simulink model "QuarterCarEKF"  (Simulink 7.5)
settings: Solver=ode45  StartTime=0.0  StopTime=5  FixedStep=0.001  MaxStep=Ts  RelTol=1e-3
PreLoadFcn:
  | QuarterCarParams
values from neighbouring files (symbols this model uses):
  actuatorDelay = 0.005    [QuarterCarParams.m]
  actuatorPole = 70    [QuarterCarParams.m]
  actuatorSat = 4000    [QuarterCarParams.m]
  g = 9.81    [QuarterCarParams.m]
  J = 1    [QuarterCarParams.m]
  Ki = 100000    [QuarterCarParams.m]
  Kp = 1200    [QuarterCarParams.m]
  lambda_ref = 0.1    [QuarterCarParams.m]
  m = 450    [QuarterCarParams.m]
  m0 = m    (= 450)    [QuarterCarParams.m]
  roadCoeffs = [1.28 23.99 0.52]    [QuarterCarParams.m]
  Ts = 0.005    [QuarterCarParams.m]
  v0 = 30    [QuarterCarParams.m]
  Wr = 0.32    [QuarterCarParams.m]
undefined symbols (not defined in the file or in its folder): DiscIntNeverNeededParam
libraries: simulink x3
settings Model: Creator=SIMONE  LastModifiedBy=Phil Goddard
settings DataIOCC: LimitDataPoints=off  SaveOutput=off  SignalLogging=off  DSMLogging=off  SaveTime=off  TimeSaveName=t_out
settings OptimizationCC: InitFltsAndDblsToZero=on
settings DebuggingCC: StrictBusMsg=Warning

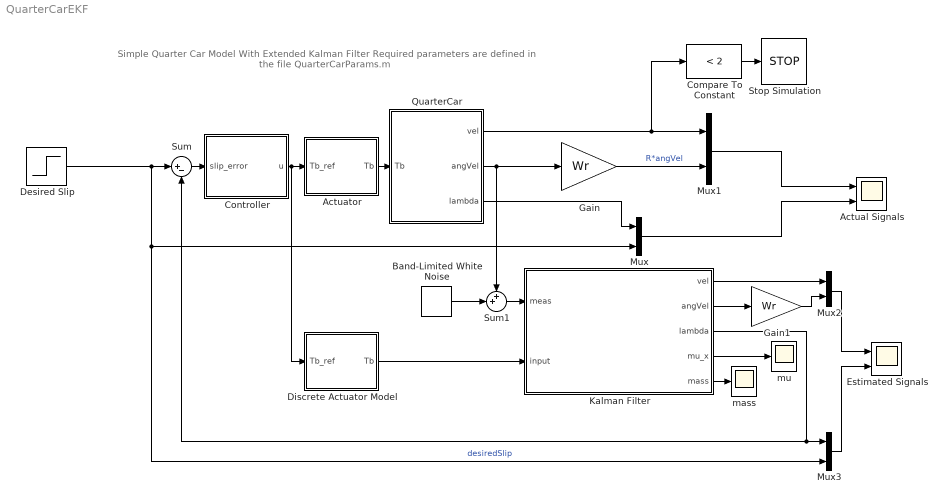
== system QuarterCarEKF ==
  note: Simple Quarter Car Model With Extended Kalman Filter
      | Required parameters are defined in the file QuarterCarParams.m
  Actual Signals : Scope  NumInputPorts=2
      settings: TimeRange=3  YMin=0~0  YMax=32~0.15
  Actuator : Subsystem  TreatAsAtomicUnit=on
      settings: MinAlgLoopOccurrences=on
  Band-Limited White Noise : simulink/Sources/Band-Limited White Noise  SystemSampleTime=-1  Cov=[0.005]  Ts=Ts  seed=[23341]
  Compare To Constant : simulink/Logic and Bit Operations/Compare To Constant  SystemSampleTime=-1  relop=<  const=2  LogicOutDataTypeMode=boolean
  Controller : Subsystem  TreatAsAtomicUnit=on  SystemSampleTime=Ts
  Desired Slip : Step  Time=0.2  After=lambda_ref  SampleTime=0
  Discrete Actuator Model : Subsystem  TreatAsAtomicUnit=on  SystemSampleTime=Ts
      settings: MinAlgLoopOccurrences=on
  Estimated Signals : Scope  NumInputPorts=2
      settings: TimeRange=3  YMin=0~0  YMax=32~0.15  SaveName=ScopeData2
  Gain : Gain  Gain=Wr  ParameterDataType=fixdt(1, 16)  ParameterScaling=2^0  OutDataType=fixdt(1, 16)  OutScaling=2^0
  Gain1 : Gain  Gain=Wr  ParameterDataType=fixdt(1, 16)  ParameterScaling=2^0  OutDataType=fixdt(1, 16)  OutScaling=2^0
  Kalman Filter : Stateflow chart  TreatAsAtomicUnit=on  SystemSampleTime=Ts
  Mux{,1..3} (4 alike) : Mux  Inputs=2
  QuarterCar : Subsystem  TreatAsAtomicUnit=on
      settings: MinAlgLoopOccurrences=on
  Stop Simulation : Stop
  Sum : Sum  Inputs=|+-  OutDataType=sfix(16)  OutScaling=2^0
  Sum1 : Sum  Inputs=++|  OutDataType=fixdt(1, 16)  OutScaling=2^0  SampleTime=Ts
  mass : Scope
      settings: TimeRange=3  YMin=449.6  YMax=450.6  SaveName=ScopeData3
  mu : Scope
      settings: TimeRange=3  YMin=-2  YMax=2  SaveName=ScopeData4
  wires:
  Controller/1(u) -> Actuator/1(Tb_ref), Discrete Actuator Model/1(Tb_ref)
  Sum/1 -> Controller/1(slip_error)
  Actuator/1(Tb) -> QuarterCar/1(Tb)
  Desired Slip/1 -> Sum/1, Mux/2, Mux3/2  "desiredSlip"
  QuarterCar/3(lambda) -> Mux/1
  QuarterCar/1(vel) -> Mux1/1, Compare To Constant/1
  QuarterCar/2(angVel) -> Gain/1, Sum1/1
  Mux1/1 -> Actual Signals/1
  Mux/1 -> Actual Signals/2
  Gain/1 -> Mux1/2  "R*angVel"
  Compare To Constant/1 -> Stop Simulation/1
  Gain1/1 -> Mux2/2
  Sum1/1 -> Kalman Filter/1(meas)
  Band-Limited White Noise/1 -> Sum1/2
  Discrete Actuator Model/1(Tb) -> Kalman Filter/2(input)
  Kalman Filter/1(vel) -> Mux2/1
  Kalman Filter/2(angVel) -> Gain1/1
  Kalman Filter/4(mu_x) -> mu/1
  Kalman Filter/5(mass) -> mass/1
  Kalman Filter/3(lambda) -> Sum/2, Mux3/1
  Mux3/1 -> Estimated Signals/2
  Mux2/1 -> Estimated Signals/1

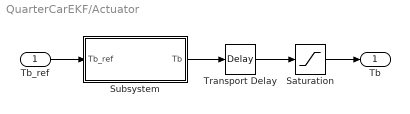
== system QuarterCarEKF/Actuator ==
  Tb_ref : Inport
  Saturation : Saturate  UpperLimit=actuatorSat  LowerLimit=0
  Subsystem : Subsystem
  Transport Delay : TransportDelay  DelayTime=actuatorDelay  BufferSize=10240
  Tb : Outport
  wires:
  Subsystem/1(Tb) -> Transport Delay/1
  Tb_ref/1 -> Subsystem/1(Tb_ref)
  Saturation/1 -> Tb/1
  Transport Delay/1 -> Saturation/1

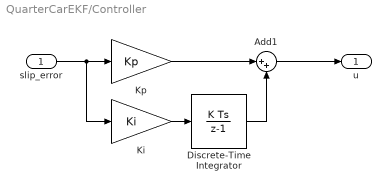
== system QuarterCarEKF/Controller ==
  slip_error : Inport  OutDataType=sfix(16)  OutScaling=2^0
  Add1 : Sum  Inputs=|++  OutDataType=sfix(16)  OutScaling=2^-10
  Discrete-Time Integrator : DiscreteIntegrator  SampleTime=-1  OutDataType=fixdt(1, 16)  OutScaling=2^0  ICPrevOutput=DiscIntNeverNeededParam  ICPrevScaledInput=DiscIntNeverNeededParam
  Ki : Gain  Gain=Ki  ParameterDataType=sfix(16)  ParameterScaling=2^0  OutDataType=sfix(16)  OutScaling=2^0
  Kp : Gain  Gain=Kp  ParameterDataType=sfix(16)  ParameterScaling=2^0  OutDataType=sfix(16)  OutScaling=2^0
  u : Outport  OutDataType=sfix(16)  OutScaling=2^0
  wires:
  slip_error/1 -> Kp/1, Ki/1
  Add1/1 -> u/1
  Kp/1 -> Add1/1
  Ki/1 -> Discrete-Time Integrator/1
  Discrete-Time Integrator/1 -> Add1/2

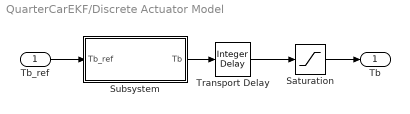
== system QuarterCarEKF/Discrete Actuator Model ==
  Tb_ref : Inport
  Saturation : Saturate  UpperLimit=actuatorSat  LowerLimit=0
  Subsystem : Subsystem
  Transport Delay : simulink/Discrete/Integer Delay  vinit=0.0  samptime=-1  NumDelays=actuatorDelay/Ts
  Tb : Outport
  wires:
  Transport Delay/1 -> Saturation/1
  Saturation/1 -> Tb/1
  Tb_ref/1 -> Subsystem/1(Tb_ref)
  Subsystem/1(Tb) -> Transport Delay/1

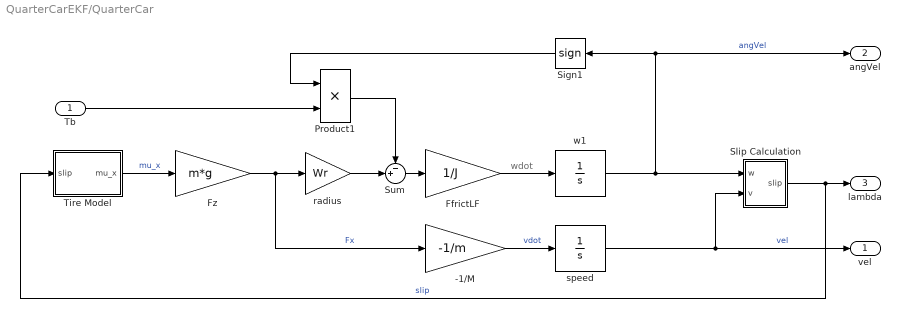
== system QuarterCarEKF/QuarterCar ==
  note: wdot
  Tb : Inport  OutDataType=sfix(16)  OutScaling=2^0
  -1/M : Gain  Gain=-1/m  ParameterDataType=sfix(16)  ParameterScaling=2^0  OutDataType=sfix(16)  OutScaling=2^0  SaturateOnIntegerOverflow=on  OutDataTypeStr=Inherit: Same as input  ParamDataTypeStr=Inherit: Same as input
  FfrictLF : Gain  Gain=1/J  ParameterDataType=sfix(16)  ParameterScaling=2^0  OutDataType=sfix(16)  OutScaling=2^0  SaturateOnIntegerOverflow=on  OutDataTypeStr=Inherit: Same as input  ParamDataTypeStr=Inherit: Same as input
  Fz : Gain  Gain=m*g  ParameterDataType=sfix(16)  ParameterScaling=2^0  OutDataType=sfix(16)  OutScaling=2^0  SaturateOnIntegerOverflow=on  OutDataTypeStr=Inherit: Same as input  ParamDataTypeStr=Inherit: Same as input
  Product1 : Product  OutDataType=sfix(16)  OutScaling=2^0  SaturateOnIntegerOverflow=on  OutDataTypeStr=Inherit: Same as first input
  Sign1 : Signum
  Slip Calculation : Subsystem
  Sum : Sum  Inputs=-+|  OutDataType=sfix(16)  OutScaling=2^0
  Tire Model : Subsystem  TreatAsAtomicUnit=on
  radius : Gain  Gain=Wr  ParameterDataType=sfix(16)  ParameterScaling=2^0  OutDataType=sfix(16)  OutScaling=2^0  SaturateOnIntegerOverflow=on  OutDataTypeStr=Inherit: Same as input  ParamDataTypeStr=Inherit: Same as input
  speed : Integrator  InitialCondition=v0  LimitOutput=on  LowerSaturationLimit=0
  w1 : Integrator  InitialCondition=v0/Wr  LimitOutput=on  LowerSaturationLimit=0
  vel : Outport  OutDataType=sfix(16)  OutScaling=2^0
  angVel : Outport  Port=2  OutDataType=sfix(16)  OutScaling=2^0
  lambda : Outport  Port=3  OutDataType=sfix(16)  OutScaling=2^0
  wires:
  -1/M/1 -> speed/1  "vdot"
  Fz/1 -> -1/M/1, radius/1  "Fx"
  Slip Calculation/1(slip) -> lambda/1, Tire Model/1(slip)  "slip"
  FfrictLF/1 -> w1/1
  Sign1/1 -> Product1/1
  Tb/1 -> Product1/2
  w1/1 -> Sign1/1, angVel/1, Slip Calculation/1(w)  "angVel"
  speed/1 -> Slip Calculation/2(v), vel/1  "vel"
  Sum/1 -> FfrictLF/1
  Tire Model/1(mu_x) -> Fz/1  "mu_x"
  radius/1 -> Sum/2
  Product1/1 -> Sum/1

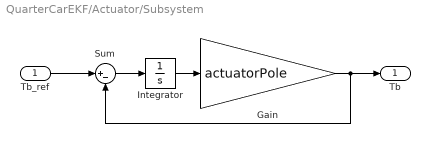
== system QuarterCarEKF/Actuator/Subsystem ==
  Tb_ref : Inport  OutDataType=fixdt(1, 16)  OutScaling=2^0
  Gain : Gain  Gain=actuatorPole  ParameterDataType=fixdt(1, 16)  ParameterScaling=2^0  OutDataType=fixdt(1, 16)  OutScaling=2^0
  Integrator : Integrator
  Sum : Sum  Inputs=|+-  OutDataType=fixdt(1, 16)  OutScaling=2^0
  Tb : Outport  OutDataType=fixdt(1, 16)  OutScaling=2^0
  wires:
  Gain/1 -> Tb/1, Sum/2
  Tb_ref/1 -> Sum/1
  Sum/1 -> Integrator/1
  Integrator/1 -> Gain/1

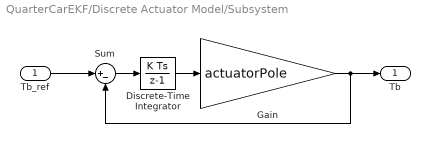
== system QuarterCarEKF/Discrete Actuator Model/Subsystem ==
  Tb_ref : Inport  OutDataType=fixdt(1, 16)  OutScaling=2^0
  Discrete-Time Integrator : DiscreteIntegrator  SampleTime=-1  OutDataType=fixdt(1, 16)  OutScaling=2^0  ICPrevOutput=DiscIntNeverNeededParam  ICPrevScaledInput=DiscIntNeverNeededParam
  Gain : Gain  Gain=actuatorPole  ParameterDataType=fixdt(1, 16)  ParameterScaling=2^0  OutDataType=fixdt(1, 16)  OutScaling=2^0
  Sum : Sum  Inputs=|+-  OutDataType=fixdt(1, 16)  OutScaling=2^0
  Tb : Outport  OutDataType=fixdt(1, 16)  OutScaling=2^0
  wires:
  Discrete-Time Integrator/1 -> Gain/1
  Sum/1 -> Discrete-Time Integrator/1
  Tb_ref/1 -> Sum/1
  Gain/1 -> Sum/2, Tb/1

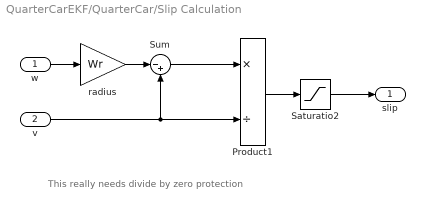
== system QuarterCarEKF/QuarterCar/Slip Calculation ==
  note: This really needs divide
      | by zero protection
  w : Inport  OutDataType=fixdt(1, 16)  OutScaling=2^0
  v : Inport  Port=2  OutDataType=fixdt(1, 16)  OutScaling=2^0
  Product1 : Product  Inputs=*/  OutDataType=sfix(16)  OutScaling=2^0  SaturateOnIntegerOverflow=on  OutDataTypeStr=Inherit: Same as first input
  Saturatio2 : Saturate  UpperLimit=1  LowerLimit=0
  Sum : Sum  Inputs=|-+  OutDataType=sfix(16)  OutScaling=2^0
  radius : Gain  Gain=Wr  ParameterDataType=sfix(16)  ParameterScaling=2^0  OutDataType=sfix(16)  OutScaling=2^0  SaturateOnIntegerOverflow=on  OutDataTypeStr=Inherit: Same as input  ParamDataTypeStr=Inherit: Same as input
  slip : Outport  OutDataType=fixdt(1, 16)  OutScaling=2^0
  wires:
  w/1 -> radius/1
  v/1 -> Sum/2, Product1/2
  radius/1 -> Sum/1
  Sum/1 -> Product1/1
  Product1/1 -> Saturatio2/1
  Saturatio2/1 -> slip/1

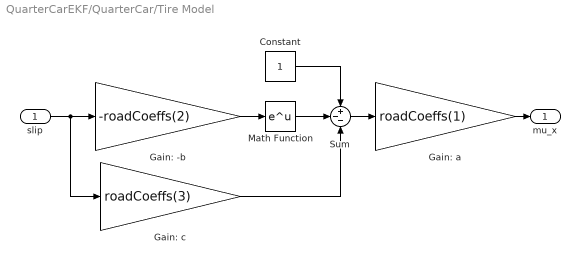
== system QuarterCarEKF/QuarterCar/Tire Model ==
  slip : Inport  OutDataType=fixdt(1, 16)  OutScaling=2^0
  Constant : Constant  OutDataType=fixdt(1, 16)  OutScaling=2^0
  Gain: -b : Gain  Gain=-roadCoeffs(2)  ParameterDataType=sfix(16)  ParameterScaling=2^0  OutDataType=sfix(16)  OutScaling=2^0  SaturateOnIntegerOverflow=on  OutDataTypeStr=Inherit: Same as input  ParamDataTypeStr=Inherit: Same as input
  Gain: a : Gain  Gain=roadCoeffs(1)  ParameterDataType=sfix(16)  ParameterScaling=2^0  OutDataType=sfix(16)  OutScaling=2^0  SaturateOnIntegerOverflow=on  OutDataTypeStr=Inherit: Same as input  ParamDataTypeStr=Inherit: Same as input
  Gain: c : Gain  Gain=roadCoeffs(3)  ParameterDataType=sfix(16)  ParameterScaling=2^0  OutDataType=sfix(16)  OutScaling=2^0  SaturateOnIntegerOverflow=on  OutDataTypeStr=Inherit: Same as input  ParamDataTypeStr=Inherit: Same as input
  Math Function : Math  OutDataType=fixdt(1, 16)  OutScaling=2^0  SaturateOnIntegerOverflow=on
  Sum : Sum  Inputs=+--  OutDataType=fixdt(1, 16)  OutScaling=2^0
  mu_x : Outport  OutDataType=fixdt(1, 16)  OutScaling=2^0
  wires:
  slip/1 -> Gain: -b/1, Gain: c/1
  Gain: -b/1 -> Math Function/1
  Math Function/1 -> Sum/2
  Constant/1 -> Sum/1
  Gain: c/1 -> Sum/3
  Sum/1 -> Gain: a/1
  Gain: a/1 -> mu_x/1

== matlab function Kalman Filter ==
  data: meas input double; input input double; vel output double; Ts parameter double; v0 parameter double; m0 parameter double; Wr parameter double; g parameter double; J parameter double; roadCoeffs parameter double; angVel output double; lambda output double; mu_x output double; mass output double
function [vel,angVel,lambda,mu_x,mass] = ...
    ExtKalman(meas,input,Ts,v0,m0,Wr,g,J,roadCoeffs)
%#eml
% This Embedded MATLAB Function implements an extended Kalman filter used
% to estimate the states, road surface and mass of a quarter car model.
%
% The states of the process are given by
% x = [omega;velocity;slip;road friction;mass];
%
% There is assumed to be one measurement
% y = [omega]
%

% Author: Phil Goddard (phil@goddardconsulting.ca)

% Define storage for the variables that need to persist
% between time periods.
persistent P xhat Q R
if isempty(P)
   % First time through the code so do some initialization
   xhat = [v0/Wr;v0;0;0;m0];
   P = zeros(5,5);
   Q = diag([0.01^2 0.01^2 1 1 0.001^2]);
   R = 0.005/Ts;
end
% Calculate the Jacobians for the state and measurement equations
F = [1 0 0 Ts*(1/J)*(Wr*g*xhat(5)) Ts*(1/J)*(Wr*g*xhat(4));
     0 1 0 Ts*(-g) 0;
     -(Wr/xhat(2)) -Wr*xhat(1) 0 0 0;
     0 0 roadCoeffs(1)*...
     (roadCoeffs(2)*exp(-roadCoeffs(2)*xhat(3))-roadCoeffs(3)) 0 0;
     0 0 0 0 1];
H = [1 0 0 0 0];
% Propogate the state and covariance matrices
xhat = [...
    xhat(1) + Ts*(1/J)*(Wr*g*xhat(4)*xhat(5) - sign(xhat(1))*input);
    xhat(2) + Ts*(-g*xhat(4));
    (xhat(2) - Wr*xhat(1))/xhat(2);
    roadCoeffs(1)*(1 - exp(-roadCoeffs(2)*xhat(3))-roadCoeffs(3)*xhat(3));
    xhat(5)];
P = F*P*F' + Q;
% Calculate the Kalman gain
K = P*H'/(H*P*H' + R);
% Calculate the measurement residual
yhat = xhat(1);
resid = meas - yhat;
% Update the state and covariance estimates
xhat = xhat + K*resid;
P = (eye(size(K,1))-K*H)*P;
% Post the results
vel = xhat(2);
angVel = xhat(1);
lambda = xhat(3);
mu_x = xhat(4);
mass = xhat(5);
